simulink model "ClassExampleMar26"  (R2018b)
settings: Solver=VariableStepAuto  StartTime=0.0  StopTime=5  RelTol=1e-3
undefined symbols (not defined in the file or in its folder): DiscIntNeverNeededParam
libraries: simulink x1
settings Model: Creator=diduch  LastModifiedBy=diduch

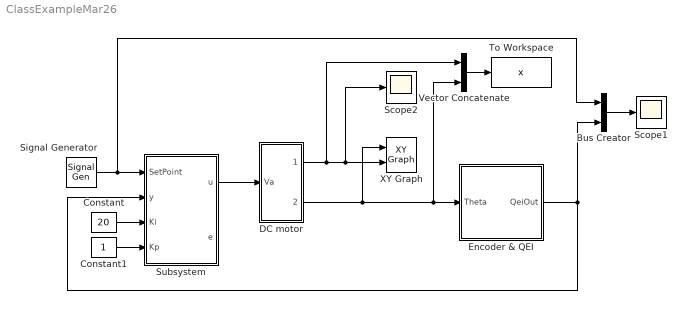
== system ClassExampleMar26 ==
  Bus Creator : BusCreator  Inputs=2
  Constant : Constant  Value=20
  Constant1 : Constant
  DC motor : Subsystem
  Encoder & QEI : Subsystem
  Scope1 : Scope
  Scope2 : Scope
  Signal Generator : SignalGenerator  WaveForm=square  Amplitude=1000  Frequency=.5
  Subsystem : Subsystem
  To Workspace : ToWorkspace  VariableName=x  SaveFormat=Timeseries  SampleTime=-1
  Vector Concatenate : Concatenate
  XY Graph : simulink/Sinks/XY Graph  xmin=-1200  xmax=1000  ymin=-2000  ymax=2000  st=-1
  wires:
  Signal Generator/1 -> Bus Creator/1, Subsystem/1(SetPoint)
  Encoder & QEI/1(QeiOut) -> Subsystem/2(y), Bus Creator/2
  DC motor/1(Omega) -> Vector Concatenate/1, Scope2/1, XY Graph/2
  DC motor/2(Theta) -> XY Graph/1, Encoder & QEI/1(Theta), Vector Concatenate/2
  Subsystem/1(u) -> DC motor/1(Va)
  Constant/1 -> Subsystem/3(Ki)
  Constant1/1 -> Subsystem/4(Kp)
  Vector Concatenate/1 -> To Workspace/1
  Bus Creator/1 -> Scope1/1

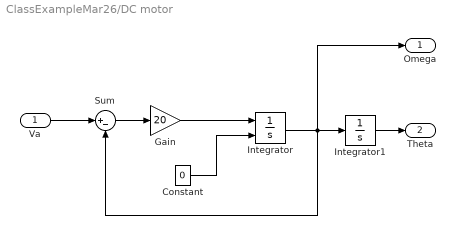
== system ClassExampleMar26/DC motor ==
  Va : Inport
  Constant : Constant  Value=0
  Gain : Gain  Gain=20
  Integrator : Integrator  InitialConditionSource=external
  Integrator1 : Integrator
  Sum : Sum  Inputs=|+-
  Omega : Outport
  Theta : Outport  Port=2
  wires:
  Gain/1 -> Integrator/1
  Constant/1 -> Integrator/2
  Va/1 -> Sum/1
  Integrator1/1 -> Theta/1
  Sum/1 -> Gain/1
  Integrator/1 -> Sum/2, Integrator1/1, Omega/1

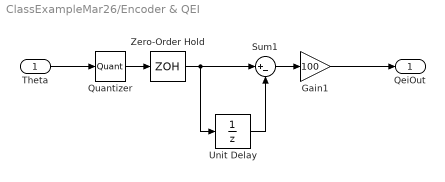
== system ClassExampleMar26/Encoder & QEI ==
  Theta : Inport
  Gain1 : Gain  Gain=100
  Quantizer : Quantizer  QuantizationInterval=2*pi/16
  Sum1 : Sum  Inputs=|+-
  Unit Delay : UnitDelay  SampleTime=0.01
  Zero-Order Hold : ZeroOrderHold  SampleTime=0.01
  QeiOut : Outport
  wires:
  Quantizer/1 -> Zero-Order Hold/1
  Zero-Order Hold/1 -> Sum1/1, Unit Delay/1
  Unit Delay/1 -> Sum1/2
  Sum1/1 -> Gain1/1
  Gain1/1 -> QeiOut/1
  Theta/1 -> Quantizer/1

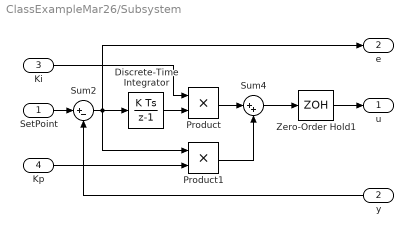
== system ClassExampleMar26/Subsystem ==
  SetPoint : Inport
  y : Inport  Port=2
  Ki : Inport  Port=3
  Kp : Inport  Port=4
  Discrete-Time Integrator : DiscreteIntegrator  SampleTime=.01  ICPrevOutput=DiscIntNeverNeededParam  ICPrevScaledInput=DiscIntNeverNeededParam
  Product : Product
  Product1 : Product
  Sum2 : Sum  Inputs=|+-
  Sum4 : Sum  Inputs=|++
  Zero-Order Hold1 : ZeroOrderHold  SampleTime=0.01
  u : Outport
  e : Outport  Port=2
  wires:
  Product1/1 -> Sum4/2
  Product/1 -> Sum4/1
  SetPoint/1 -> Sum2/1
  Zero-Order Hold1/1 -> u/1
  Sum2/1 -> e/1, Product1/1, Discrete-Time Integrator/1
  Discrete-Time Integrator/1 -> Product/2
  y/1 -> Sum2/2
  Sum4/1 -> Zero-Order Hold1/1
  Kp/1 -> Product1/2
  Ki/1 -> Product/1
